simulink model "sim3"  (R2023a)
settings: Solver=VariableStepAuto  StartTime=0  StopTime=100  RelTol=1e-8
undefined symbols (not defined in the file): in_sw, ki, kp, reg_sw
settings Model: Creator=vasil  LastModifiedBy=vasil

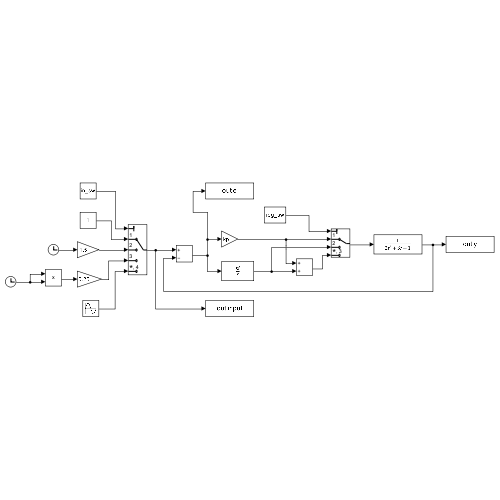
[thumbnail: Simulink's stored preview of the top-level diagram]
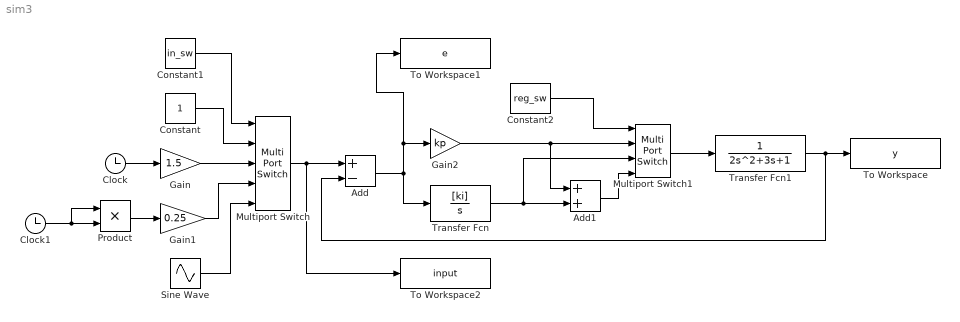
== system sim3 ==
  Add : Sum  Inputs=+-
  Add1 : Sum
  Clock : Clock
      settings: Decimation=t_end
  Clock1 : Clock
      settings: Decimation=t_end
  Constant : Constant
  Constant1 : Constant  Value=in_sw
  Constant2 : Constant  Value=reg_sw
  Gain : Gain  Gain=1.5
  Gain1 : Gain  Gain=0.25
  Gain2 : Gain  Gain=kp
  Multiport Switch : MultiPortSwitch  Inputs=4  SaturateOnIntegerOverflow=off  InputSameDT=off
  Multiport Switch1 : MultiPortSwitch  SaturateOnIntegerOverflow=off  InputSameDT=off
  Product : Product
  Sine Wave : Sin  Frequency=0.25  SampleTime=0
  To Workspace : ToWorkspace  VariableName=y  SaveFormat=Timeseries  SampleTime=-1
  To Workspace1 : ToWorkspace  VariableName=e  SaveFormat=Timeseries  SampleTime=-1
  To Workspace2 : ToWorkspace  VariableName=input  SaveFormat=Timeseries  SampleTime=-1
  Transfer Fcn : TransferFcn  Numerator=[ki]  Denominator=[1 0]
  Transfer Fcn1 : TransferFcn  Denominator=[2 3 1]
  wires:
  Constant/1 -> Multiport Switch/2
  Constant1/1 -> Multiport Switch/1
  Gain/1 -> Multiport Switch/3
  Clock/1 -> Gain/1
  Gain1/1 -> Multiport Switch/4
  Product/1 -> Gain1/1
  Clock1/1 -> Product/1, Product/2
  Sine Wave/1 -> Multiport Switch/5
  Multiport Switch/1 -> To Workspace2/1, Add/1
  Add/1 -> To Workspace1/1, Gain2/1, Transfer Fcn/1
  Gain2/1 -> Multiport Switch1/2, Add1/1
  Transfer Fcn/1 -> Add1/2, Multiport Switch1/3
  Add1/1 -> Multiport Switch1/4
  Constant2/1 -> Multiport Switch1/1
  Transfer Fcn1/1 -> Add/2, To Workspace/1
  Multiport Switch1/1 -> Transfer Fcn1/1
